simulink model "bci_1d_horizontal_control_current_system_adaptive"  (R2013a)
settings: Solver=ode45  StartTime=0.0  StopTime=Inf  FixedStep=1  RelTol=1e-3
InitFcn:
  | clc
  | firstAttempt = true;
  | fs = 125;
  | phase = 1;%horizontal phase
  | 
  | if(firstAttempt)%linear regression model with all features on
  | 
  | eegSession = Csv2BciStruct('db\bci_users\matanga_ny\phase1\matanga_ny_phase1_07062016_9h28pm.csv');
  | [restClass,leftClass] = eegSessionGroupClasses(eegSession);
  | AllClass = [restClass leftClass];
  | NTrials = length(AllClass);
  | %Channels Selection
  | ChannelList =[7,10,12,14,16,21,24];
  | 
  | %Features Extraction
  | p = 16;
  | bandSize = 4;
  | uFreq = 40;
  | for i=1:NTrials
  | eeg = eegStruct2Array(AllClass(i));
  | eegOut = eeg(:,ChannelList);
  | Bands = eegARmodel(eegOut,p,bandSize,uFreq,fs);%NBands x NCh
  | %Feature Selection
  | Features = [Bands(8,1) Bands(5,2)  Bands(3,3) Bands(4,3) Bands(6,3) Bands(7,3) ...
  |     Bands(8,3)  Bands(10,3) Bands(11,3)  Bands(5,4) Bands(6,4)...
  |     Bands(8,4) Bands(9,4) Bands(8,5) Bands(3,6) Bands(8,6) ...
  |     Bands(3,7) Bands(8,7) ];
  | F(i,:) = Features;
  | end
  | %model parameters
  | NFr = size(F,2);
  | beta_x = [0 ones(1,NFr)];
  | DX = mlr_regressor(beta_x',F);
  | 
  | %normalization parameters estimation
  | [mean_dx,std_dx]=zscore_norm(DX);
  | 
  | val = [beta_x,mean_dx,std_dx];
  | disp('...MLR :initial model....')
  | 
  | else
  | 
  | load('db\bci_users\matanga_ny\phase1_5\matanga_ny_phase1.5_2_6_2016_15h50.mat');
  | beta_x = modelParametersBundle{end};
  | stats = statsBundle{end};
  | mean_dx = stats(1);
  | std_dx =stats(2);
  | val = [beta_x,mean_dx,std_dx];
  | disp('...MLR : start model....')
  | 
  | end
  | 
  | valString = strcat('[',num2str(val),']');
  | set_param('bci_1d_horizontal_control_current_system_adaptive/model_parameters','Value',valString);
model workspace (MAT data in the model file):
  local_ip = 2130706433
  local_port = 50224
  host_ip = 2130706433
  host_port = 50223
  serial_number = 'NB-2014.07.69'
  sample_rate = 250
  num_samples = 8
  num_en_channels = 32
  en_add_channels = 5
  cfg_native : struct (value not decoded)
undefined symbols (not defined in the file): get, NB
libraries: dspnetwork x3, dspsnks4 x2, simulink x1, gNautilusLib x1
PauseFcn:
  | fs = 125;
  | BufferLength = 10;%10 previous trials
  | Nsd = 13;
  | phase = 1;%horizontal phase
  | 
  | [F,D] = getTrainingSetsMLR(sim_out,BufferLength,phase,Nsd);
  | 
  | if ~isempty(F)
  | 
  | tic
  | disp('LS-MLR Training ....')
  | [beta_x] = lsmlr(F,D);
  | toc
  | 
  | Dx = mlr_regressor(beta_x,F);
  | R2 = R2coef(F,D,Dx);
  | %normalization parameters estimation
  | [mean_dx,std_dx]=zscore_norm(Dx);
  | 
  | val = [beta_x' mean_dx std_dx];
  | disp('.......... LSMLR Parameter :...')
  | beta_x
  | disp('....... Normalization .....:....')
  | mean_dx
  | std_dx
  | disp('..... Goodness of fit ...........')
  | R2
  | valString = strcat('[',num2str(val),']');
  | set_param('bci_1d_horizontal_control_current_system_adaptive/model_parameters','Value',valString);
  | disp('...MLR : update model....')
  | 
  | else
  | 
  | disp('... No Data Found To Train The Model...')
  | 
  | end
  | %resume simulation
  | set_param('bci_1d_horizontal_control_current_system_adaptive','SimulationCommand','continue'),
  | disp('... Resume simulation...')
settings Model: Creator=Yves Matanga  LastModifiedBy=Yves Matanga
settings SolverCC: ZeroCrossControl=EnableAll

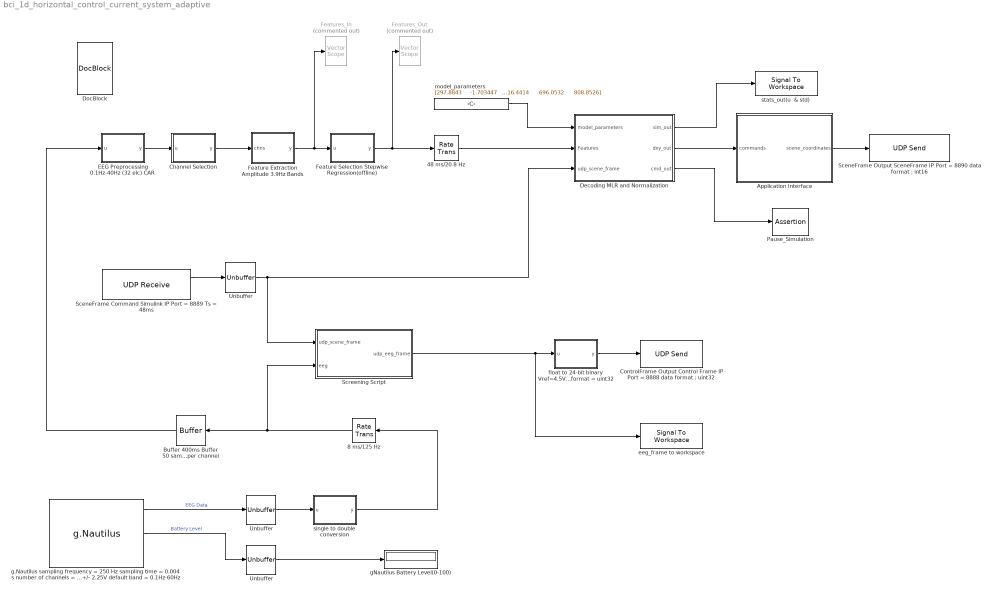
== system bci_1d_horizontal_control_current_system_adaptive ==
  " 48 ms/20.8 Hz " : RateTransition  OutPortSampleTime=0.048
  8 ms/125 Hz : RateTransition  OutPortSampleTime=0.008
  Application Interface : MATLAB Function  TreatAsAtomicUnit=on  SystemSampleTime=0.048
  Buffer 400ms Buffer 50 samples per channel : Buffer  N=50  V=49  TreatMby1Signals=One channel
  Channel Selection : MATLAB Function  TreatAsAtomicUnit=on  SystemSampleTime=0.008
  "ControlFrame Output Control Frame IP Port = 8888 data format : uint32" : dspnetwork/UDP Send  remoteURL='168.172.200.69'  remotePort=8888  localURL='0.0.0.0'  localPortSource=Automatically determine  localPort=-1  sampletime=-1  separateLengthPort=0
  Decoding MLR and Normalization : MATLAB Function  TreatAsAtomicUnit=on  SystemSampleTime=0.048
  DocBlock : simulink/Model-Wide Utilities/DocBlock  DocumentType=Text
      content=|
      | The Above platform is for EEG capturing a
      | and samping of screening imagery .
      |
      | A JAVA GUI is running aside this simulink and communicate
      | via UDP protocol
      |
      | Once the Screening start ,the Java scene GUI send a start
      | command to the simulink model (ASCII for '1' ) which
      | will trigger a sampling signal to 1
      |
      | Once the Screening stopped ,the Java GUI will send a stop command
      | to the simulink model (ASCII for '2') which will trigger
      | a sampling signal to 2
      |
      | else it iso 0
      |
      | the sampling signal will help extract the eeg signals of the
      | user motor imagery ,hence
      |
      | the interval between a start (1) and a stop (2) is
      | basically "a single trial eeg imagery"
      |
      | all the eeg signals will be transferred at all time to the java
      | application which save into a database for furhter recovery.
      |
      | Note that all blocks must have the sampling time as dictated by the EEG source
      | T = 0.004s (250Hz)
      |
      | ---------------------------------------------------------------------------------------------------------
      | UPDATES :
      |
      | (*) Target Number Reception Included (From JAVA SceneControlPanel)
      | (*) Training From N (10 = default) previous trials datasets very well now(with variable size)
      |
      | Problems :
      |
      | (*) How To Update Previous BCI weights to the current one
      |     Make Sure You Save Them in The Database for later use
      | (*) Output Normalization Must not be based upon the previous feature only because (they can be an error in the
      |     previous trial)
      | (*) Is There A Real Need for input Normalization ????
      | (*) How To Take Care of Nan in Features because they disrupt the feature set selection process
      |
      | Solution :
      |
      | (*) May be you can discard trials with Nan Features  ---> Just Make Sure To Count How Many
      | They are to see if it is really relevant
  EEG Preprocessing 0.1Hz-40Hz (32 elc) CAR : MATLAB Function  TreatAsAtomicUnit=on  SystemSampleTime=0.008
  Feature Extraction Amplitude 3.9Hz Bands : MATLAB Function  TreatAsAtomicUnit=on  SystemSampleTime=0.008
  Feature Selection Stepwise Regression(offline) : MATLAB Function  TreatAsAtomicUnit=on  SystemSampleTime=0.008
  Features_In : dspsnks4/Vector Scope  Commented=on  ScopeProperties=on  Domain=User-defined  HorizSpan=1  DisplayProperties=off  AxisGrid=on  Memory=off  FrameNumber=on  AxisLegend=on  AxisZoom=off  OpenScopeAtSimStart=on  OpenScopeImmediately=off  FigPos=get(0,'defaultfigureposition')  AxisProperties=off  XUnits=Hertz  XRange=[0...Fs/2]  InheritXIncr=on  XIncr=1  XLabel=Frequency Bands (0 :2:40 Hz)  XLimit=Auto  XMin=0  XMax=40  XStart=0  YUnits=dB  YLabel=Amplitude  LineProperties=off  LineStyles=:|:  LineMarkers=stem|stem|.|x  LineColors=[1 0 0]|[0 1 0]|[0 1 1]  XAxisParamsVer=6.9
      settings: YMin=-10  YMax=10
  Features_Out : dspsnks4/Vector Scope  Commented=on  ScopeProperties=on  Domain=User-defined  HorizSpan=1  DisplayProperties=off  AxisGrid=on  Memory=off  FrameNumber=on  AxisLegend=on  AxisZoom=off  OpenScopeAtSimStart=on  OpenScopeImmediately=off  FigPos=get(0,'defaultfigureposition')  AxisProperties=off  XUnits=Hertz  XRange=[0...Fs/2]  InheritXIncr=on  XIncr=1  XLabel=Frequency Bands (0 :2:40 Hz)  XLimit=Auto  XMin=0  XMax=40  XStart=0  YUnits=dB  YLabel=Amplitude  LineProperties=off  LineStyles=:|:  LineMarkers=stem|stem|.|x  LineColors=[1 0 0]|[0 1 0]|[0 1 1]  XAxisParamsVer=6.9
      settings: YMin=-10  YMax=10
  Pause_Simulation : Assertion  AssertionFailFcn=|  StopWhenAssertionFail=off  SampleTime=0.048
      | set_param(bdroot,'SimulationCommand','pause'),
      | disp(sprintf('\nSimulation paused.'))
  SceneFrame Command Simulink IP Port = 8889 Ts = 48ms : dspnetwork/UDP Receive  localURL='0.0.0.0'  localPort=8889  remoteURL='168.172.200.69'  remotePort=-1  recvBufferSize=8192  dims=255  signalDatatype=uint8  isVarSize=off  showBlockingTime=off  blockingTime=0  sampletime=0.048
  "SceneFrame Output SceneFrame IP Port = 8890 data format : int16" : dspnetwork/UDP Send  remoteURL='168.172.200.69'  remotePort=8890  localURL='0.0.0.0'  localPortSource=Automatically determine  localPort=-1  sampletime=-1  separateLengthPort=0
  Screening Script : MATLAB Function  TreatAsAtomicUnit=on  SystemSampleTime=0.008
  Unbuffer : Unbuffer  SampleBasedProcessing=Same as frame based
  "Unbuffer " : Unbuffer  SampleBasedProcessing=Same as frame based
  "Unbuffer   " : Unbuffer  SampleBasedProcessing=Same as frame based
  eeg_frame to workspace : SignalToWorkspace  VariableName=eeg_frame
      settings: CopyFcn=dspblkcopystw(gcbh);
  float to 24-bit binary Vref=4.5V(in uV) Mean = 2.25V data format = uint32 : MATLAB Function  TreatAsAtomicUnit=on  SystemSampleTime=0.008
  "g.Nautilus sampling frequency = 250 Hz sampling time = 0.004 s number of channels = 32 resolution = 24 Bit output = float32 unit = uV dynamic range = +/- 2.25V default band = 0.1Hz-60Hz " : gNautilusLib/g.Nautilus  Tag=g.Nautilus  Description=Operates a g.Nautilus device and provides acquired data on its outputs.  sample_rate=250  local_ip=2130706433  local_port=50224  host_ip=2130706433  host_port=50223  serial_number=NB-2014.07.69  num_samples=8  num_en_channels=32  add_channels=5
  gNautilus Battery Level(0-100) : Display
  model_parameters : Constant  Value="[297.8843     -1.703447      40.93116      79.78982      41.00967       46.8178     -55.23426      138.6526      27.16669      87.51416     -147.4492      3.130156     -142.3237     -12.07293      14.86169      41.85342     -31.46488     -99.82819      116.4414      696.0532      808.8526]"  SampleTime=-1
  single to double conversion : MATLAB Function  TreatAsAtomicUnit=on  SystemSampleTime=0.004
  stats_out(u  & std) : SignalToWorkspace  VariableName=sim_out
      settings: CopyFcn=dspblkcopystw(gcbh);
  wires:
  "g.Nautilus sampling frequency = 250 Hz sampling time = 0.004 s number of channels = 32 resolution = 24 Bit output = float32 unit = uV dynamic range = +/- 2.25V default band = 0.1Hz-60Hz "/1 -> Unbuffer/1  "EEG Data"
  Unbuffer/1 -> single to double conversion/1(u)
  SceneFrame Command Simulink IP Port = 8889 Ts = 48ms/1 -> "Unbuffer "/1
  8 ms/125 Hz/1 -> Buffer 400ms Buffer 50 samples per channel/1, Screening Script/2(eeg)
  float to 24-bit binary Vref=4.5V(in uV) Mean = 2.25V data format = uint32/1(y) -> "ControlFrame Output Control Frame IP Port = 8888 data format : uint32"/1
  single to double conversion/1(y) -> 8 ms/125 Hz/1
  Feature Extraction Amplitude 3.9Hz Bands/1(y) -> Feature Selection Stepwise Regression(offline)/1(u), Features_In/1
  Screening Script/1(udp_eeg_frame) -> float to 24-bit binary Vref=4.5V(in uV) Mean = 2.25V data format = uint32/1(u), eeg_frame to workspace/1
  Channel Selection/1(y) -> Feature Extraction Amplitude 3.9Hz Bands/1(chns)
  EEG Preprocessing 0.1Hz-40Hz (32 elc) CAR/1(y) -> Channel Selection/1(u)
  Application Interface/1(scene_coordinates) -> "SceneFrame Output SceneFrame IP Port = 8890 data format : int16"/1
  "Unbuffer   "/1 -> gNautilus Battery Level(0-100)/1
  Decoding MLR and Normalization/2(dxy_out) -> Application Interface/1(commands)
  "Unbuffer "/1 -> Decoding MLR and Normalization/3(udp_scene_frame), Screening Script/1(udp_scene_frame)
  "g.Nautilus sampling frequency = 250 Hz sampling time = 0.004 s number of channels = 32 resolution = 24 Bit output = float32 unit = uV dynamic range = +/- 2.25V default band = 0.1Hz-60Hz "/2 -> "Unbuffer   "/1  "Battery Level"
  Buffer 400ms Buffer 50 samples per channel/1 -> EEG Preprocessing 0.1Hz-40Hz (32 elc) CAR/1(u)
  Feature Selection Stepwise Regression(offline)/1(y) -> " 48 ms/20.8 Hz "/1, Features_Out/1
  " 48 ms/20.8 Hz "/1 -> Decoding MLR and Normalization/2(Features)
  Decoding MLR and Normalization/1(sim_out) -> stats_out(u  & std)/1
  model_parameters/1 -> Decoding MLR and Normalization/1(model_parameters)
  Decoding MLR and Normalization/3(cmd_out) -> Pause_Simulation/1

== matlab function bci_1d_horizontal_control_current_system_adaptive/single to double conversion ==
  data: u input; y output
function y = fcn(u)
%#codegen
y = double(u);

== matlab function bci_1d_horizontal_control_current_system_adaptive/Screening Script ==
  data: udp_scene_frame input; eeg input; udp_eeg_frame output
function udp_eeg_frame  = fcn( udp_scene_frame,eeg)
%#codegen
 if udp_scene_frame == uint8('1') %START in ASCII
     udp_eeg_frame = [eeg 1];%timing frame = 1
 elseif udp_scene_frame == uint8('2') %STOP
     udp_eeg_frame = [eeg 2];%timing frame = 2
 else
     udp_eeg_frame = [eeg 0];%timing frame = 0
 end
 
 %the purpose of this function to 
 %save the  eeg signals sampled with the start
 %and stop of every trial%

== matlab function bci_1d_horizontal_control_current_system_adaptive/EEG Preprocessing 0.1Hz-40Hz (32 elc) CAR ==
  data: u input; y output
function y = fcn(u)
%Input EEG (0.1Hz - 60Hz) with 50Hz Notch
%Preprocessing Stage (0.1Hz - 40Hz) Signal 
%fHigh = 40;% 40Hz
%fs = 250;%250Hz
%order = 5 ;% Filter Order
%[bw,aw] = butter(order,[fHigh]/(fs/2));%Butterworth filter
%yf = filter(bw,aw,u);%filtered ( < 40Hz)
%y = eegHjorthSL(u);%Surface Laplacian 
%(Large Laplacian : Must Be Small Laplacian as you're using 32 electrodes)
y = eegCarf(u);%Common Average

== matlab function bci_1d_horizontal_control_current_system_adaptive/float to 24-bit binary Vref=4.5V(in uV) Mean = 2.25V data format = uint32 ==
  data: u input; y output
function y = fcn(u)
 eeg_frame = u(1:32);
 %convert to 24 bit binary
 bin = uint32((eeg_frame + 2.25e6)*(2^24-1)/(4.5e6));
y = [bin uint32(u(33))]; %Select All Channels

== matlab function bci_1d_horizontal_control_current_system_adaptive/Channel Selection ==
  data: u input; y output
function y = fcn(u)
%#codegen

%channel lookup table
% 1 --  FP1                      % 17 --  C4
% 2 --  FP2                      % 18 --  T8
% 3 --  AF3                      % 19 --  CP5
% 4 --  AF4                      % 20 --  CP1
% 5 --  F7                       % 21 --  CP2
% 6 --  F3                       % 22 --  CP6
% 7 --  FZ                       % 23 --  P7 
% 8 --  F4                       % 24 --  P3
% 9 --  F8                       % 25 --  PZ
% 10 -- FC5                      % 26 --  P4
% 11 -- FC1                      % 27 --  P8
% 12 -- FC2                      % 28 --  PO7
% 13 -- FC6                      % 29 --  PO3
% 14 -- T7                       % 30 --  PO4
% 15 -- C3                       % 31 --  PO8
% 16 -- CZ                       % 32 --  OZ

Ch = [7,10,12,14,16,21,24];
y = u(:,Ch); %Select All Channels

== matlab function bci_1d_horizontal_control_current_system_adaptive/Feature Extraction Amplitude 3.9Hz Bands ==
  data: chns input; y output
function y = fcn(chns)
%Input : NSamplesxChannels
%Autoregressive Model (16th Order ) : Burg Algorithm
p = 16;
bandSize = 4;%3Hz BandSize
fs = 125;%sampling frequency
uFreq = 40;%40Hz
y = eegARmodel(chns,p,bandSize,uFreq,fs);%NBands x NCh

== matlab function bci_1d_horizontal_control_current_system_adaptive/Application Interface ==
  data: commands input; scene_coordinates output
function scene_coordinates  = fcn(commands)
%#codegen
% persistent dy;
% step = 1;%pixel setp
% screenHeight = 1018;
% if isempty(dy)
%     dy = -3*screenHeight/8;
% end
%sending daa via UDP
scene_coordinates = [int16(commands(1)) int16(commands(2))];
%dy = dy + step;%cursor moving up in y direction...

== matlab function bci_1d_horizontal_control_current_system_adaptive/Feature Selection Stepwise Regression(offline) ==
  data: u input; y output
function y = fcn(u)
%features selection
%features_Ids = [4 6 13 14];
% y = [u(8,1) u(5,2) u(2,3) u(3,3) u(4,3) u(6,3) u(7,3) ...
%     u(8,3) u(9,3) u(10,3) u(11,3) u(3,4) u(5,4) u(6,4)...
%     u(8,4) u(9,4) u(8,5) u(3,6) u(8,6) u(1,7) u(2,7)...
%     u(3,7) u(8,7) u(9,7)];

y = [u(8,1) u(5,2)  u(3,3) u(4,3) u(6,3) u(7,3) ...
    u(8,3)  u(10,3) u(11,3)  u(5,4) u(6,4)...
    u(8,4) u(9,4) u(8,5) u(3,6) u(8,6) ...
    u(3,7) u(8,7) ];

== matlab function bci_1d_horizontal_control_current_system_adaptive/Decoding MLR and Normalization ==
  data: model_parameters input; sim_out output; dxy_out output; Features input; udp_scene_frame input; cmd_out output
function [sim_out,dxy_out,cmd_out] = fcn(model_parameters,Features,udp_scene_frame)
%variable declarations
persistent beta_x;%regression coefficients (MLR) [1xNCoeffs]
persistent target_id;%position of target in scenario
persistent mean_dx;
persistent std_dx;
persistent dy;
persistent cmd;


gain = 10;%15*screenHeight*3/(8*Nht);%with a slow moving cursor

if (isempty(target_id)||isempty(beta_x))%by deault consider target 1
    target_id=1;
   beta_x = model_parameters(1:end-2);
   mean_dx = model_parameters(end-1); 
   std_dx = model_parameters(end);
   dy =  3;
   cmd = 1;
end
dxy = zeros(1,2);
dxy_raw = zeros(1,2);
%trainging time
if ~isempty(find(udp_scene_frame==uint8('1')))%start of paradigm       
    sync = 1;
    trial_on = true;    
    cmd = 1;
elseif ~isempty(find(udp_scene_frame==uint8('2'))) %STOP PRACTICE       
    sync = 2; 
    cmd = 0;%pause simulation to retrain
elseif ~isempty(find((udp_scene_frame >=uint8('3')) & ...
        (udp_scene_frame <=uint8('6')) ))%target number received
    sync = 0;
    target_id= double(udp_scene_frame(1)-48-2);    
    cmd = 1;
else
    sync = 0;%for timing of data
    cmd = 1;
end
%real time regression
beta_x = model_parameters(1:end-2);
mean_dx = model_parameters(end-1); 
std_dx = model_parameters(end);    
dxy_raw(1) =  mlr_regressor(beta_x,Features); 
dxy_raw(2) = dy;
%output normalization
dxy(1) = gain*zscore(dxy_raw(1),mean_dx,std_dx);%normalize output
dxy(2) = dxy_raw(2);
%append sync to facilitate data removal
dxy_out = dxy;
sim_out = [beta_x' mean_dx std_dx dxy dxy_raw Features target_id sync];
%simulation commands
cmd_out = cmd;
